simulink model "EKF_Sim_MLE"  (R2018a)
settings: Solver=ode4  StartTime=0  StopTime=time_end  FixedStep=time_step  MaxStep=0.1  RelTol=1e-15  AbsTol=1e-15
values from neighbouring files (symbols this model uses):
  mu = 398600.4418    [FFNAV_EKF_STM.m]
  N_window = 30    [FFNAV_EKF_MLE_Run.m]
  time_step = 1    [FFNAV_EKF_MLE_Run.m]
undefined symbols (not defined in the file or in its folder): a_chaser, a_target, AoP_chaser, AoP_target, e_chaser, e_target, GPS_r_STD, GPS_v_STD, i_chaser, i_target, n, Q0, R0, RAAN_chaser, RAAN_target, theta0_chaser, theta0_target
libraries: dspindex x2
settings Model: Creator=corytfraser  LastModifiedBy=Cory
settings SolverCC: AutoScaleAbsTol=off
settings DataIOCC: LimitDataPoints=on  SaveFormat=Array  SignalLoggingSaveFormat=ModelDataLogs
settings OptimizationCC: BlockReduction=off  BooleanDataType=off  ExpressionDepthLimit=2147483647  LifeSpan=inf
settings DebuggingCC: SaveWithParameterizedLinksMsg=none  UnderspecifiedInitializationDetection=Classic  MergeDetectMultiDrivingBlocksExec=none  SignalResolutionControl=TryResolveAllWithWarning  MultiTaskDSMMsg=warning  MultiTaskCondExecSysMsg=none  FcnCallInpInsideContextMsg=warning  AllowSymbolicDim=off  StateNameClashWarn=warning  SFUnexpectedBacktrackingDiag=warning  SFNoUnconditionalDefaultTransitionDiag=warning  SFExecutionAtInitializationDiag=none
settings HardwareCC: ProdBitPerPointer=32  ProdBitPerSizeT=32  ProdBitPerPtrDiffT=32  ProdLargestAtomicFloat=None  ProdIntDivRoundTo=Undefined  ProdEndianess=Unspecified  ProdWordSize=32  ProdHWDeviceType=32-bit Generic  TargetUnknown=on
settings ModelReferenceCC: PropagateSignalLabelsOutOfModel=off
settings CodeAppCC: StateflowObjectComments=on
settings GRTTargetCC: TargetLangStandard=C89/C90 (ANSI)  GeneratePreprocessorConditionals=Disable all
settings ConfigComp: CovMetricSettings=dw  CovHtmlReporting=on  CovSaveCumulativeToWorkspaceVar=on  CovSaveSingleToWorkspaceVar=on  CovExternalEMLEnable=off  CovSFcnEnable=off

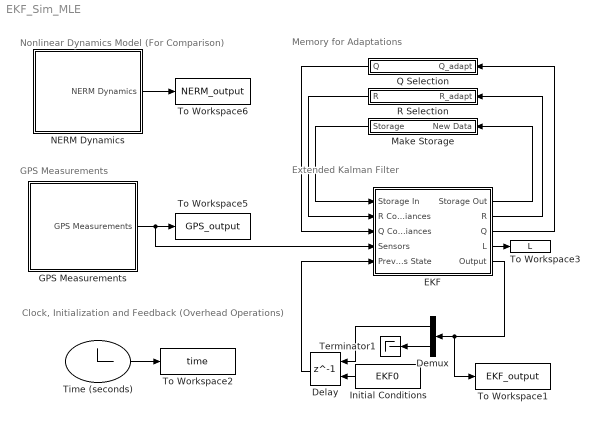
== system EKF_Sim_MLE ==
  note: Memory for Adaptations
  note: Clock, Initialization and Feedback (Overhead Operations)
  note: Extended Kalman Filter
  note: GPS Measurements
  note: Nonlinear Dynamics Model (For Comparison)
  Delay : Delay  DelayLength=1  InitialConditionSource=Input port  InitialCondition=0  SampleTime=time_step
      settings: InputPortMap=u0,p4
  Demux : Demux  Outputs=[117 -1]
  EKF : Subsystem
  "GPS Measurements " : Subsystem
      mask Display: image('C:\Users\Cory\OneDrive\FFNAV Project\MATLAB Code\NERM EKF Simulation\Masks\GPS Image.jpg');
  Initial Conditions : FromWorkspace  VariableName=EKF0  SampleTime=time_step
  Make Storage : Subsystem
  NERM Dynamics : Subsystem
      mask Display: image('C:\Users\Cory\OneDrive\FFNAV Project\MATLAB Code\NERM EKF Simulation\Masks\Proba-3.jpg');
  Q Selection : Subsystem
  R Selection : Subsystem
  Terminator1 : Terminator
  Time (seconds) : Clock
  To Workspace1 : ToWorkspace  VariableName=EKF_output  SampleTime=-1
  To Workspace2 : ToWorkspace  VariableName=time  SampleTime=-1
  To Workspace3 : ToWorkspace  VariableName=L  SampleTime=-1
  To Workspace5 : ToWorkspace  VariableName=GPS_output  SampleTime=-1
  To Workspace6 : ToWorkspace  VariableName=NERM_output  SampleTime=-1
  wires:
  Time (seconds)/1 -> To Workspace2/1
  Demux/1 -> Delay/1
  NERM Dynamics/1(NERM Dynamics) -> To Workspace6/1
  Initial Conditions/1 -> Delay/2
  Delay/1 -> EKF/5(Previous State)
  Demux/2 -> Terminator1/1
  EKF/4(L) -> To Workspace3/1
  "GPS Measurements "/1(GPS Measurements) -> EKF/4(Sensors), To Workspace5/1
  EKF/3(Q) -> Q Selection/1(Q_adapt)
  Q Selection/1(Q) -> EKF/3(Q Covariances)
  EKF/2(R) -> R Selection/1(R_adapt)
  R Selection/1(R) -> EKF/2(R Covariances)
  EKF/5(Output) -> Demux/1, To Workspace1/1
  EKF/1(Storage Out) -> Make Storage/1(New Data)
  Make Storage/1(Storage) -> EKF/1(Storage In)

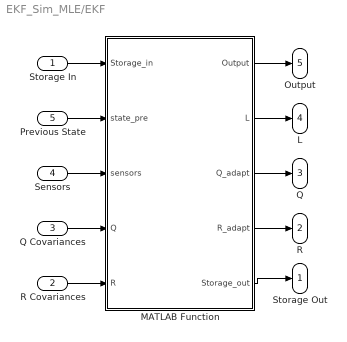
== system EKF_Sim_MLE/EKF ==
  Storage In : Inport
  R Covariances : Inport  Port=2
  Q Covariances : Inport  Port=3
  Sensors : Inport  Port=4
  Previous State : Inport  Port=5
  MATLAB Function : MATLAB Function  TreatAsAtomicUnit=on
  Storage Out : Outport
  R : Outport  Port=2
  Q : Outport  Port=3
  L : Outport  Port=4
  Output : Outport  Port=5
  wires:
  MATLAB Function/1(Output) -> Output/1
  Previous State/1 -> MATLAB Function/2(state_pre)
  Q Covariances/1 -> MATLAB Function/4(Q)
  R Covariances/1 -> MATLAB Function/5(R)
  Sensors/1 -> MATLAB Function/3(sensors)
  MATLAB Function/2(L) -> L/1
  MATLAB Function/3(Q_adapt) -> Q/1
  MATLAB Function/4(R_adapt) -> R/1
  MATLAB Function/5(Storage_out) -> Storage Out/1
  Storage In/1 -> MATLAB Function/1(Storage_in)

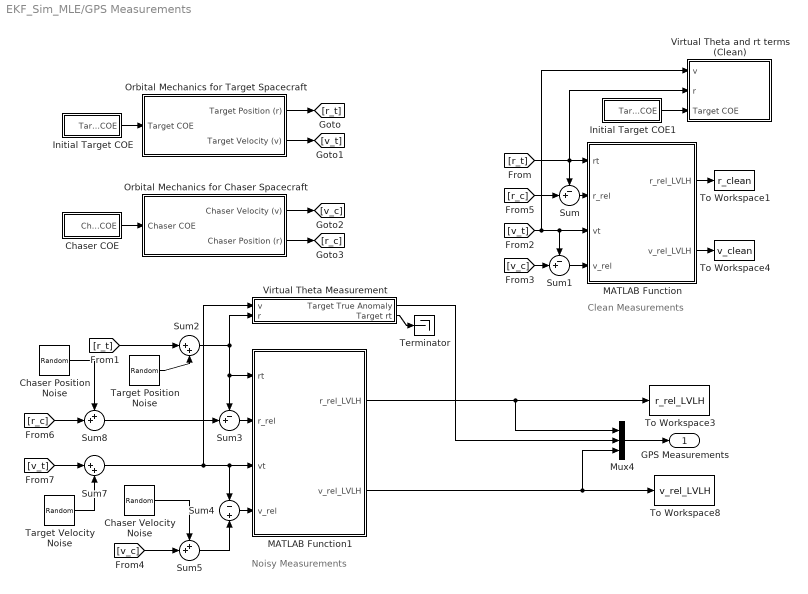
== system EKF_Sim_MLE/GPS Measurements  ==
  note: Noisy Measurements
  note: Clean Measurements
  Chaser COE : Subsystem
  Chaser Position Noise : RandomNumber  Variance=GPS_r_STD^2  Seed=1222  SampleTime=time_step
  Chaser Velocity Noise : RandomNumber  Variance=GPS_v_STD^2  Seed=99999999  SampleTime=time_step
  Initial Target COE : Subsystem
  Initial Target COE1 : Subsystem
  MATLAB Function : MATLAB Function  TreatAsAtomicUnit=on
  MATLAB Function1 : MATLAB Function  TreatAsAtomicUnit=on
  Mux4 : Mux  Inputs=3
  Orbital Mechanics for Target Spacecraft : Subsystem
  Orbital Mechanics for Chaser Spacecraft : Subsystem
  Sum : Sum  Inputs=-+|
  Sum1 : Sum  Inputs=-+|
  Sum2 : Sum  Inputs=|++
  Sum3 : Sum  Inputs=-+|
  Sum4 : Sum  Inputs=-|+
  Sum5 : Sum  Inputs=++|
  Sum7 : Sum  Inputs=|++
  Sum8 : Sum  Inputs=++|
  Target Position Noise : RandomNumber  Variance=GPS_r_STD^2  Seed=999  SampleTime=time_step
  Target Velocity Noise : RandomNumber  Variance=GPS_v_STD^2  Seed=2000  SampleTime=time_step
  Terminator : Terminator
  To Workspace1 : ToWorkspace  VariableName=r_clean  SampleTime=-1
  To Workspace3 : ToWorkspace  VariableName=r_rel_LVLH  SampleTime=-1
  To Workspace4 : ToWorkspace  VariableName=v_clean  SampleTime=-1
  To Workspace8 : ToWorkspace  VariableName=v_rel_LVLH  SampleTime=-1
  Virtual Theta Measurement : Subsystem
  Virtual Theta and rt terms (Clean) : Subsystem
  GPS Measurements : Outport
  wires:
  Orbital Mechanics for Target Spacecraft/1(Target Position (r)) -> [r_t]
  Sum/1 -> MATLAB Function/2(r_rel)
  Sum1/1 -> MATLAB Function/4(v_rel)
  MATLAB Function/2(v_rel_LVLH) -> To Workspace4/1
  MATLAB Function/1(r_rel_LVLH) -> To Workspace1/1
  Mux4/1 -> GPS Measurements/1
  Initial Target COE/1(Target COE) -> Orbital Mechanics for Target Spacecraft/1(Target COE)
  Chaser COE/1(Chaser COE) -> Orbital Mechanics for Chaser Spacecraft/1(Chaser COE)
  MATLAB Function1/2(v_rel_LVLH) -> Mux4/3, To Workspace8/1
  MATLAB Function1/1(r_rel_LVLH) -> Mux4/1, To Workspace3/1
  Sum7/1 -> Virtual Theta Measurement/1(v), MATLAB Function1/3(vt), Sum4/1
  Sum3/1 -> MATLAB Function1/2(r_rel)
  Sum4/1 -> MATLAB Function1/4(v_rel)
  Sum5/1 -> Sum4/2
  Sum8/1 -> Sum3/2
  [r_t] -> Virtual Theta and rt terms (Clean)/2(r), MATLAB Function/1(rt), Sum/1
  [v_t] -> Virtual Theta and rt terms (Clean)/1(v), Sum1/1, MATLAB Function/3(vt)
  [v_c] -> Sum1/2
  Orbital Mechanics for Chaser Spacecraft/1(Chaser Velocity (v)) -> [v_c]
  [r_c] -> Sum/2
  Orbital Mechanics for Chaser Spacecraft/2(Chaser Position (r)) -> [r_c]
  Orbital Mechanics for Target Spacecraft/2(Target Velocity (v)) -> [v_t]
  [r_t] -> Sum2/1
  [r_c] -> Sum8/2
  [v_t] -> Sum7/1
  [v_c] -> Sum5/2
  Sum2/1 -> MATLAB Function1/1(rt), Sum3/1, Virtual Theta Measurement/2(r)
  Chaser Position Noise/1 -> Sum8/1
  Target Position Noise/1 -> Sum2/2
  Target Velocity Noise/1 -> Sum7/2
  Chaser Velocity Noise/1 -> Sum5/1
  Initial Target COE1/1(Target COE) -> Virtual Theta and rt terms (Clean)/3(Target COE)
  Virtual Theta Measurement/1(Target True Anomaly) -> Mux4/2
  Virtual Theta Measurement/2(Target rt) -> Terminator/1

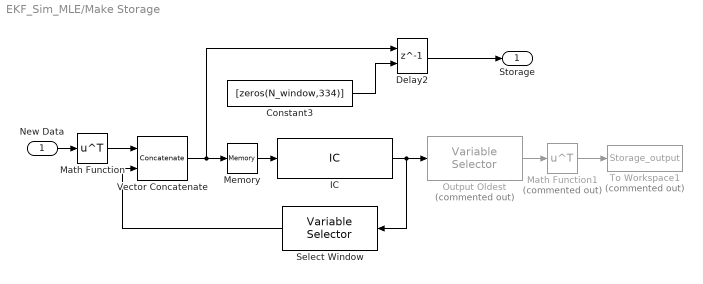
== system EKF_Sim_MLE/Make Storage ==
  New Data : Inport
  Constant3 : Constant  Value=[zeros(N_window,334)]
  Delay2 : Delay  DelayLength=1  InitialConditionSource=Input port  InitialCondition=0  SampleTime=time_step
      settings: InputPortMap=u0,p4
  IC : InitialCondition  Value=[zeros(N_window,334)]
  Math Function : Math  Operator=transpose  SaturateOnIntegerOverflow=on
  Math Function1 : Math  Commented=on  Operator=transpose  SaturateOnIntegerOverflow=on
  Memory : Memory
  Output Oldest : dspindex/Variable Selector  Commented=on  NumInputs=1  rowsOrCols=Rows  IdxMode=Fixed  Elements=N_window  ZerOneIdxMode=One-based  errmode=Clip Index  FillMode=on  FillValues=0
  Select Window : dspindex/Variable Selector  NumInputs=1  rowsOrCols=Rows  IdxMode=Fixed  Elements=1:N_window-1  ZerOneIdxMode=One-based  errmode=Clip Index  FillMode=on  FillValues=0
  To Workspace1 : ToWorkspace  Commented=on  VariableName=Storage_output  SampleTime=-1
  Vector Concatenate : Concatenate  Mode=Multidimensional array
  Storage : Outport
  wires:
  IC/1 -> Output Oldest/1, Select Window/1
  Memory/1 -> IC/1
  Select Window/1 -> Vector Concatenate/2
  New Data/1 -> Math Function/1
  Vector Concatenate/1 -> Delay2/1, Memory/1
  Math Function/1 -> Vector Concatenate/1
  Delay2/1 -> Storage/1
  Constant3/1 -> Delay2/2
  Math Function1/1 -> To Workspace1/1
  Output Oldest/1 -> Math Function1/1

== system EKF_Sim_MLE/NERM Dynamics ==
  Demux : Demux  Outputs=[10 -1]
  Demux1 : Demux  Outputs=10
  Initial Conditions : FromWorkspace  VariableName=EKF0  SampleTime=time_step
  Mux : Mux  Inputs=10
  NERM Propagation : Subsystem
  Terminator1 : Terminator
  NERM Dynamics : Outport
  wires:
  Demux1/9 -> NERM Propagation/9(theta_dot0)
  Demux1/6 -> NERM Propagation/6(x_dot0_chaser)
  Demux1/10 -> NERM Propagation/10(rt_dot0)
  Demux1/4 -> NERM Propagation/4(theta0_target)
  Demux1/3 -> NERM Propagation/3(z0_chaser)
  Initial Conditions/1 -> Demux/1
  Demux1/7 -> NERM Propagation/7(y_dot0_chaser)
  Demux1/2 -> NERM Propagation/2(y0_chaser)
  Demux1/1 -> NERM Propagation/1(x0_chaser)
  NERM Propagation/1(x) -> Mux/1
  Demux1/5 -> NERM Propagation/5(rt0)
  NERM Propagation/2(y) -> Mux/2
  NERM Propagation/3(z) -> Mux/3
  Demux/1 -> Demux1/1  "Initial  State Vector"
  NERM Propagation/7(y_dot) -> Mux/7
  NERM Propagation/4(theta_target) -> Mux/4
  NERM Propagation/9(theta_dot_target) -> Mux/9
  NERM Propagation/10(rt_dot) -> Mux/10
  NERM Propagation/6(x_dot) -> Mux/6
  NERM Propagation/8(z_dot) -> Mux/8
  NERM Propagation/5(rt) -> Mux/5
  Demux1/8 -> NERM Propagation/8(z_dot0_chaser)
  Mux/1 -> NERM Dynamics/1
  Demux/2 -> Terminator1/1

== system EKF_Sim_MLE/Q Selection ==
  Q_adapt : Inport
  Constant2 : Constant  Value=Q0
  Delay1 : Delay  DelayLength=1  InitialConditionSource=Input port  InitialCondition=0  SampleTime=time_step
      settings: InputPortMap=u0,p4
  Switch: Q Adaptation On/Off : ManualSwitch
  To Workspace4 : ToWorkspace  VariableName=Q_output  SampleTime=-1
  Q : Outport
  wires:
  Switch: Q Adaptation On/Off/1 -> Delay1/1
  Constant2/1 -> Switch: Q Adaptation On/Off/2, Delay1/2
  Q_adapt/1 -> Switch: Q Adaptation On/Off/1
  Delay1/1 -> To Workspace4/1, Q/1

== system EKF_Sim_MLE/R Selection ==
  R_adapt : Inport
  Constant3 : Constant  Value=R0
  Delay2 : Delay  DelayLength=1  InitialConditionSource=Input port  InitialCondition=0  SampleTime=time_step
      settings: InputPortMap=u0,p4
  Switch: R Adaptation On/Off : ManualSwitch
  To Workspace7 : ToWorkspace  VariableName=R_output  SampleTime=-1
  R : Outport
  wires:
  Switch: R Adaptation On/Off/1 -> Delay2/1
  Constant3/1 -> Switch: R Adaptation On/Off/2, Delay2/2
  Delay2/1 -> R/1, To Workspace7/1
  R_adapt/1 -> Switch: R Adaptation On/Off/1

== system EKF_Sim_MLE/GPS Measurements /Chaser COE ==
  Argument of Perigee (w)1 : Constant  Value=AoP_chaser
  Eccentricity (e)1 : Constant  Value=e_chaser
  Inclination (i)1 : Constant  Value=i_chaser
  Mux1 : Mux  Inputs=6
  RAAN (Omega)1 : Constant  Value=RAAN_chaser
  Semi-Major Axis (a)1 : Constant  Value=a_chaser
  True Anomaly (theta) : Constant  Value=theta0_chaser
  Chaser COE : Outport
  wires:
  Mux1/1 -> Chaser COE/1
  Argument of Perigee (w)1/1 -> Mux1/6
  True Anomaly (theta)/1 -> Mux1/1
  Semi-Major Axis (a)1/1 -> Mux1/2
  Inclination (i)1/1 -> Mux1/4
  RAAN (Omega)1/1 -> Mux1/5
  Eccentricity (e)1/1 -> Mux1/3

== system EKF_Sim_MLE/GPS Measurements /Initial Target COE ==
  Argument of Perigee (w) : Constant  Value=AoP_target
  Eccentricity (e) : Constant  Value=e_target
  Inclination (i) : Constant  Value=i_target
  Mux : Mux  Inputs=6
  RAAN (Omega) : Constant  Value=RAAN_target
  Semi-Major Axis (a) : Constant  Value=a_target
  Target True Anomaly (theta) : Constant  Value=theta0_target
  Target COE : Outport
  wires:
  Argument of Perigee (w)/1 -> Mux/6
  RAAN (Omega)/1 -> Mux/5
  Eccentricity (e)/1 -> Mux/3
  Semi-Major Axis (a)/1 -> Mux/2
  Target True Anomaly (theta)/1 -> Mux/1
  Inclination (i)/1 -> Mux/4
  Mux/1 -> Target COE/1

== system EKF_Sim_MLE/GPS Measurements /Initial Target COE1 ==
  Argument of Perigee (w) : Constant  Value=AoP_target
  Eccentricity (e) : Constant  Value=e_target
  Inclination (i) : Constant  Value=i_target
  Mux : Mux  Inputs=6
  RAAN (Omega) : Constant  Value=RAAN_target
  Semi-Major Axis (a) : Constant  Value=a_target
  Target True Anomaly (theta) : Constant  Value=theta0_target
  Target COE : Outport
  wires:
  Argument of Perigee (w)/1 -> Mux/6
  RAAN (Omega)/1 -> Mux/5
  Eccentricity (e)/1 -> Mux/3
  Semi-Major Axis (a)/1 -> Mux/2
  Target True Anomaly (theta)/1 -> Mux/1
  Inclination (i)/1 -> Mux/4
  Mux/1 -> Target COE/1

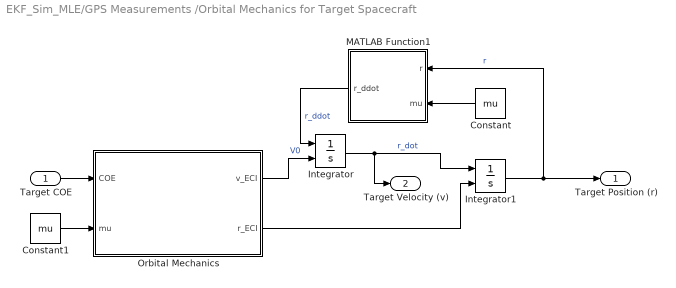
== system EKF_Sim_MLE/GPS Measurements /Orbital Mechanics for Target Spacecraft ==
  Target COE : Inport
  Constant : Constant  Value=mu
  Constant1 : Constant  Value=mu
  Integrator : Integrator  InitialConditionSource=external
  Integrator1 : Integrator  InitialConditionSource=external
  MATLAB Function1 : MATLAB Function  TreatAsAtomicUnit=on
  Orbital Mechanics : MATLAB Function  TreatAsAtomicUnit=on
  Target Position (r) : Outport
  Target Velocity (v) : Outport  Port=2
  wires:
  Integrator/1 -> Target Velocity (v)/1, Integrator1/1  "r_dot"
  MATLAB Function1/1(r_ddot) -> Integrator/1  "r_ddot"
  Integrator1/1 -> Target Position (r)/1, MATLAB Function1/1(r)  "r"
  Orbital Mechanics/2(r_ECI) -> Integrator1/2
  Orbital Mechanics/1(v_ECI) -> Integrator/2  "V0"
  Target COE/1 -> Orbital Mechanics/1(COE)
  Constant/1 -> MATLAB Function1/2(mu)
  Constant1/1 -> Orbital Mechanics/2(mu)

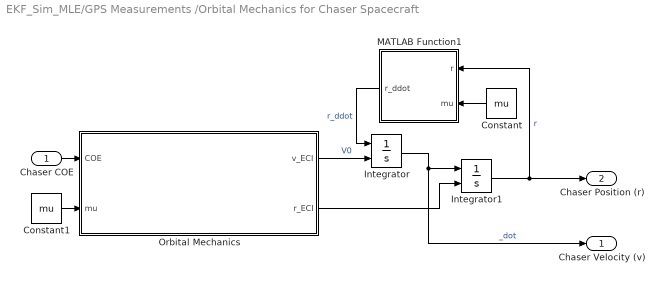
== system EKF_Sim_MLE/GPS Measurements /Orbital Mechanics for Chaser Spacecraft ==
  Chaser COE : Inport
  Constant : Constant  Value=mu
  Constant1 : Constant  Value=mu
  Integrator : Integrator  InitialConditionSource=external
  Integrator1 : Integrator  InitialConditionSource=external
  MATLAB Function1 : MATLAB Function  TreatAsAtomicUnit=on
  Orbital Mechanics : MATLAB Function  TreatAsAtomicUnit=on
  Chaser Velocity (v) : Outport
  Chaser Position (r) : Outport  Port=2
  wires:
  Integrator/1 -> Chaser Velocity (v)/1, Integrator1/1  "_dot"
  MATLAB Function1/1(r_ddot) -> Integrator/1  "r_ddot"
  Integrator1/1 -> MATLAB Function1/1(r), Chaser Position (r)/1  "r"
  Orbital Mechanics/2(r_ECI) -> Integrator1/2
  Orbital Mechanics/1(v_ECI) -> Integrator/2  "V0"
  Chaser COE/1 -> Orbital Mechanics/1(COE)
  Constant/1 -> MATLAB Function1/2(mu)
  Constant1/1 -> Orbital Mechanics/2(mu)

== system EKF_Sim_MLE/GPS Measurements /Virtual Theta Measurement ==
  v : Inport
  r : Inport  Port=2
  Constant3 : Constant  Value=theta0_target
  Integrator2 : Integrator  InitialConditionSource=external
  MATLAB Function2 : MATLAB Function  TreatAsAtomicUnit=on
  To Workspace5 : ToWorkspace  VariableName=theta_target  SampleTime=-1
  Target True Anomaly : Outport
  Target rt : Outport  Port=2
  wires:
  r/1 -> MATLAB Function2/1(r)
  Integrator2/1 -> Target True Anomaly/1, To Workspace5/1
  MATLAB Function2/1(theta_dot) -> Integrator2/1
  Constant3/1 -> Integrator2/2
  v/1 -> MATLAB Function2/2(v)
  MATLAB Function2/2(rt) -> Target rt/1

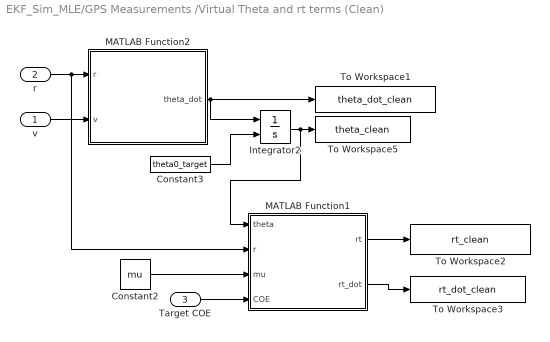
== system EKF_Sim_MLE/GPS Measurements /Virtual Theta and rt terms (Clean) ==
  v : Inport
  r : Inport  Port=2
  Target COE : Inport  Port=3
  Constant2 : Constant  Value=mu
  Constant3 : Constant  Value=theta0_target
  Integrator2 : Integrator  InitialConditionSource=external
  MATLAB Function1 : MATLAB Function  TreatAsAtomicUnit=on
  MATLAB Function2 : MATLAB Function  TreatAsAtomicUnit=on
  To Workspace1 : ToWorkspace  VariableName=theta_dot_clean  SampleTime=-1
  To Workspace2 : ToWorkspace  VariableName=rt_clean  SampleTime=-1
  To Workspace3 : ToWorkspace  VariableName=rt_dot_clean  SampleTime=-1
  To Workspace5 : ToWorkspace  VariableName=theta_clean  SampleTime=-1
  wires:
  r/1 -> MATLAB Function1/2(r), MATLAB Function2/1(r)
  Integrator2/1 -> MATLAB Function1/1(theta), To Workspace5/1
  MATLAB Function2/1(theta_dot) -> Integrator2/1, To Workspace1/1
  Constant3/1 -> Integrator2/2
  v/1 -> MATLAB Function2/2(v)
  MATLAB Function1/1(rt) -> To Workspace2/1
  MATLAB Function1/2(rt_dot) -> To Workspace3/1
  Target COE/1 -> MATLAB Function1/4(COE)
  Constant2/1 -> MATLAB Function1/3(mu)

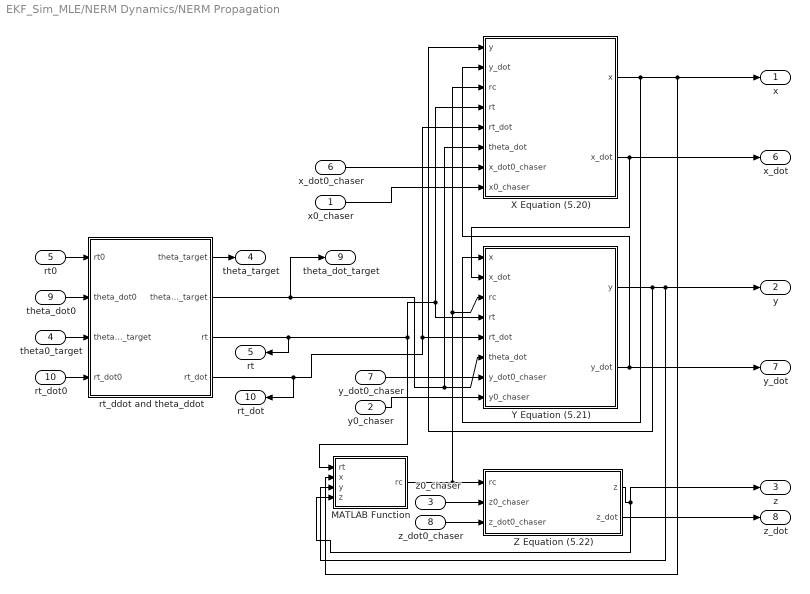
== system EKF_Sim_MLE/NERM Dynamics/NERM Propagation ==
  x0_chaser : Inport
  y0_chaser : Inport  Port=2
  z0_chaser : Inport  Port=3
  theta0_target : Inport  Port=4
  rt0 : Inport  Port=5
  x_dot0_chaser : Inport  Port=6
  y_dot0_chaser : Inport  Port=7
  z_dot0_chaser : Inport  Port=8
  theta_dot0 : Inport  Port=9
  rt_dot0 : Inport  Port=10
  MATLAB Function : MATLAB Function  TreatAsAtomicUnit=on
  X Equation (5.20) : Subsystem
  Y Equation (5.21) : Subsystem
  Z Equation (5.22) : Subsystem
  rt_ddot and theta_ddot : Subsystem
  x : Outport
  y : Outport  Port=2
  z : Outport  Port=3
  theta_target : Outport  Port=4
  rt : Outport  Port=5
  x_dot : Outport  Port=6
  y_dot : Outport  Port=7
  z_dot : Outport  Port=8
  theta_dot_target : Outport  Port=9
  rt_dot : Outport  Port=10
  wires:
  MATLAB Function/1(rc) -> X Equation (5.20)/3(rc), Y Equation (5.21)/3(rc), Z Equation (5.22)/1(rc)
  rt_ddot and theta_ddot/4(rt_dot) -> X Equation (5.20)/5(rt_dot), Y Equation (5.21)/5(rt_dot), rt_dot/1
  Y Equation (5.21)/2(y_dot) -> y_dot/1, X Equation (5.20)/2(y_dot)
  X Equation (5.20)/2(x_dot) -> x_dot/1, Y Equation (5.21)/2(x_dot)
  rt_ddot and theta_ddot/2(theta_dot_target) -> theta_dot_target/1, X Equation (5.20)/6(theta_dot), Y Equation (5.21)/6(theta_dot)
  rt_ddot and theta_ddot/3(rt) -> Y Equation (5.21)/4(rt), X Equation (5.20)/4(rt), MATLAB Function/1(rt), rt/1
  X Equation (5.20)/1(x) -> x/1, MATLAB Function/2(x), Y Equation (5.21)/1(x)
  Y Equation (5.21)/1(y) -> y/1, MATLAB Function/3(y), X Equation (5.20)/1(y)
  Z Equation (5.22)/1(z) -> MATLAB Function/4(z), z/1
  rt0/1 -> rt_ddot and theta_ddot/1(rt0)
  theta_dot0/1 -> rt_ddot and theta_ddot/2(theta_dot0)
  y_dot0_chaser/1 -> Y Equation (5.21)/7(y_dot0_chaser)
  y0_chaser/1 -> Y Equation (5.21)/8(y0_chaser)
  x0_chaser/1 -> X Equation (5.20)/8(x0_chaser)
  x_dot0_chaser/1 -> X Equation (5.20)/7(x_dot0_chaser)
  z0_chaser/1 -> Z Equation (5.22)/2(z0_chaser)
  z_dot0_chaser/1 -> Z Equation (5.22)/3(z_dot0_chaser)
  theta0_target/1 -> rt_ddot and theta_ddot/3(theta0_target)
  rt_dot0/1 -> rt_ddot and theta_ddot/4(rt_dot0)
  Z Equation (5.22)/2(z_dot) -> z_dot/1
  rt_ddot and theta_ddot/1(theta_target) -> theta_target/1

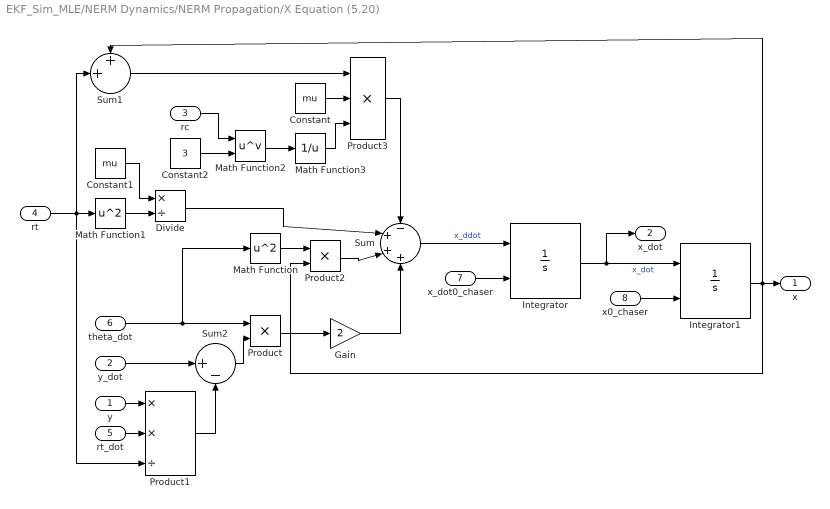
== system EKF_Sim_MLE/NERM Dynamics/NERM Propagation/X Equation (5.20) ==
  y : Inport
  y_dot : Inport  Port=2
  rc : Inport  Port=3
  rt : Inport  Port=4
  rt_dot : Inport  Port=5
  theta_dot : Inport  Port=6
  x_dot0_chaser : Inport  Port=7
  x0_chaser : Inport  Port=8
  Constant : Constant  Value=mu
  Constant1 : Constant  Value=mu
  Constant2 : Constant  Value=3
  Divide : Product  Inputs=*/
  Gain : Gain  Gain=2
  Integrator : Integrator  InitialConditionSource=external
  Integrator1 : Integrator  InitialConditionSource=external
  Math Function : Math  Operator=square  SaturateOnIntegerOverflow=on
  Math Function1 : Math  Operator=square  SaturateOnIntegerOverflow=on
  Math Function2 : Math  Operator=pow  SaturateOnIntegerOverflow=on
  Math Function3 : Math  Operator=reciprocal  SaturateOnIntegerOverflow=on
  Product : Product
  Product1 : Product  Inputs=**/
  Product2 : Product
  Product3 : Product  Inputs=3
  Sum : Sum  Inputs=-+++
  Sum1 : Sum  Inputs=++|
  Sum2 : Sum  Inputs=|+-
  x : Outport
  x_dot : Outport  Port=2
  wires:
  Sum/1 -> Integrator/1  "x_ddot"
  Integrator/1 -> Integrator1/1, x_dot/1  "x_dot"
  x_dot0_chaser/1 -> Integrator/2
  Constant/1 -> Product3/2
  Integrator1/1 -> Product2/2, Sum1/1, x/1
  rc/1 -> Math Function2/1
  x0_chaser/1 -> Integrator1/2
  rt/1 -> Sum1/2, Product1/3, Math Function1/1
  Sum1/1 -> Product3/1
  Constant1/1 -> Divide/1
  Divide/1 -> Sum/2
  Product/1 -> Gain/1
  theta_dot/1 -> Product/1, Math Function/1
  y_dot/1 -> Sum2/1
  y/1 -> Product1/1
  rt_dot/1 -> Product1/2
  Product1/1 -> Sum2/2
  Sum2/1 -> Product/2
  Math Function/1 -> Product2/1
  Product2/1 -> Sum/3
  Gain/1 -> Sum/4
  Math Function1/1 -> Divide/2
  Constant2/1 -> Math Function2/2
  Math Function2/1 -> Math Function3/1
  Math Function3/1 -> Product3/3
  Product3/1 -> Sum/1

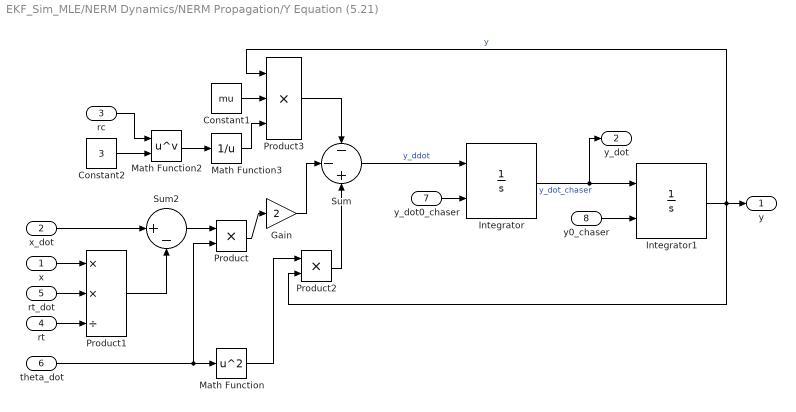
== system EKF_Sim_MLE/NERM Dynamics/NERM Propagation/Y Equation (5.21) ==
  x : Inport
  x_dot : Inport  Port=2
  rc : Inport  Port=3
  rt : Inport  Port=4
  rt_dot : Inport  Port=5
  theta_dot : Inport  Port=6
  y_dot0_chaser : Inport  Port=7
  y0_chaser : Inport  Port=8
  Constant1 : Constant  Value=mu
  Constant2 : Constant  Value=3
  Gain : Gain  Gain=2
  Integrator : Integrator  InitialConditionSource=external
  Integrator1 : Integrator  InitialConditionSource=external
  Math Function : Math  Operator=square  SaturateOnIntegerOverflow=on
  Math Function2 : Math  Operator=pow  SaturateOnIntegerOverflow=on
  Math Function3 : Math  Operator=reciprocal  SaturateOnIntegerOverflow=on
  Product : Product
  Product1 : Product  Inputs=**/
  Product2 : Product
  Product3 : Product  Inputs=3
  Sum : Sum  Inputs=--+
  Sum2 : Sum  Inputs=|+-
  y : Outport
  y_dot : Outport  Port=2
  wires:
  y_dot0_chaser/1 -> Integrator/2
  y0_chaser/1 -> Integrator1/2
  Integrator/1 -> y_dot/1, Integrator1/1  "y_dot_chaser"
  Sum/1 -> Integrator/1  "y_ddot"
  Integrator1/1 -> Product2/2, Product3/1, y/1  "y"
  Product/1 -> Gain/1
  theta_dot/1 -> Product/2, Math Function/1
  Product1/1 -> Sum2/2
  Math Function/1 -> Product2/1
  Gain/1 -> Sum/2
  Product2/1 -> Sum/3
  x_dot/1 -> Sum2/1
  x/1 -> Product1/1
  rt_dot/1 -> Product1/2
  rt/1 -> Product1/3
  Sum2/1 -> Product/1
  Constant1/1 -> Product3/2
  rc/1 -> Math Function2/1
  Constant2/1 -> Math Function2/2
  Math Function2/1 -> Math Function3/1
  Math Function3/1 -> Product3/3
  Product3/1 -> Sum/1

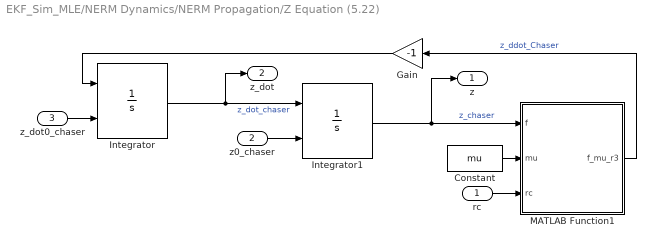
== system EKF_Sim_MLE/NERM Dynamics/NERM Propagation/Z Equation (5.22) ==
  rc : Inport
  z0_chaser : Inport  Port=2
  z_dot0_chaser : Inport  Port=3
  Constant : Constant  Value=mu
  Gain : Gain  Gain=-1
  Integrator : Integrator  InitialConditionSource=external
  Integrator1 : Integrator  InitialConditionSource=external
  MATLAB Function1 : MATLAB Function  TreatAsAtomicUnit=on
  z : Outport
  z_dot : Outport  Port=2
  wires:
  Constant/1 -> MATLAB Function1/2(mu)
  Integrator/1 -> z_dot/1, Integrator1/1  "z_dot_chaser"
  Integrator1/1 -> z/1, MATLAB Function1/1(f)  "z_chaser"
  Gain/1 -> Integrator/1
  MATLAB Function1/1(f_mu_r3) -> Gain/1  "z_ddot_Chaser"
  z_dot0_chaser/1 -> Integrator/2
  z0_chaser/1 -> Integrator1/2
  rc/1 -> MATLAB Function1/3(rc)

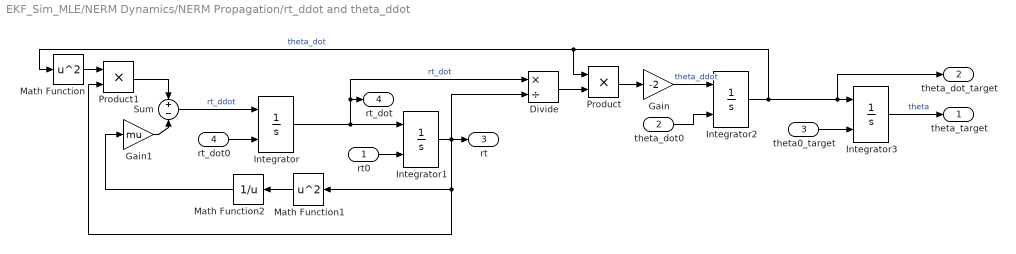
== system EKF_Sim_MLE/NERM Dynamics/NERM Propagation/rt_ddot and theta_ddot ==
  rt0 : Inport
  theta_dot0 : Inport  Port=2
  theta0_target : Inport  Port=3
  rt_dot0 : Inport  Port=4
  Divide : Product  Inputs=*/
  Gain : Gain  Gain=-2
  Gain1 : Gain  Gain=mu
  Integrator : Integrator  InitialConditionSource=external
  Integrator1 : Integrator  InitialConditionSource=external
  Integrator2 : Integrator  InitialConditionSource=external  InitialCondition=n
  Integrator3 : Integrator  InitialConditionSource=external
  Math Function : Math  Operator=square  SaturateOnIntegerOverflow=on
  Math Function1 : Math  Operator=square  SaturateOnIntegerOverflow=on
  Math Function2 : Math  Operator=reciprocal  SaturateOnIntegerOverflow=on
  Product : Product
  Product1 : Product
  Sum : Sum  Inputs=+|-
  theta_target : Outport
  theta_dot_target : Outport  Port=2
  rt : Outport  Port=3
  rt_dot : Outport  Port=4
  wires:
  Gain1/1 -> Sum/2
  Math Function2/1 -> Gain1/1
  Math Function1/1 -> Math Function2/1
  Math Function/1 -> Product1/1
  Integrator3/1 -> theta_target/1  "theta"
  Product/1 -> Gain/1
  Sum/1 -> Integrator/1  "rt_ddot"
  Integrator2/1 -> Integrator3/1, theta_dot_target/1, Math Function/1, Product/1  "theta_dot"
  Integrator1/1 -> Product1/2, Math Function1/1, Divide/2, rt/1
  Integrator/1 -> Integrator1/1, Divide/1, rt_dot/1  "rt_dot"
  Divide/1 -> Product/2
  Gain/1 -> Integrator2/1  "theta_ddot"
  theta0_target/1 -> Integrator3/2
  rt_dot0/1 -> Integrator/2
  rt0/1 -> Integrator1/2
  Product1/1 -> Sum/1
  theta_dot0/1 -> Integrator2/2

== matlab function EKF_Sim_MLE/GPS Measurements /Orbital Mechanics for Target Spacecraft/MATLAB Function1 ==
  data: r input; r_ddot output; mu input
function r_ddot = r_ddot(r, mu)
% ========================================================================
% Description: This function calculates -mu/r^3 *r to propagate the radius
% vector of the orbital motion

r_ddot = -(mu/(norm(r))^3)*r;

end
% ========================================================================

== matlab function EKF_Sim_MLE/GPS Measurements /Orbital Mechanics for Target Spacecraft/Orbital Mechanics ==
  data: v_ECI output; COE input; r_ECI output; mu input
 function [v_ECI,r_ECI] = Orb_Mech(COE, mu)
% ========================================================================
% Description: This funciton calculates the initial r and v vectors, 
% given the provided classiclal orbital elements defined in the
% initialization of the simulation.

%%========================================================================
%Extract COE values
theta       = COE(1);
a           = COE(2);
e           = COE(3);
i           = COE(4);
RAAN        = COE(5);
w           = COE(6);

%%========================================================================
r   = a*(1-e^2)/(1+e*cos(theta));                               %Defining the radius (Eq. 2.32)
p   = a*(1-e^2);                                                %Defining the semilatus rectum (Eq. 2.31)
r_P = [r*cos(theta) r*sin(theta) 0]';                           %(r in perifocal frame - Eq. 2.86) 
v_P = [-sqrt(mu/p)*sin(theta) sqrt(mu/p)*(e+cos(theta)) 0]';    %(v in perifocal frame - Eq. 2.87)

%Rotation Matrix from P to ECI Frame
C_IP = [    cos(RAAN)*cos(w)-sin(RAAN)*cos(i)*sin(w) -cos(RAAN)*sin(w)-sin(RAAN)*cos(i)*cos(w) sin(RAAN)*sin(i);
            sin(RAAN)*cos(w)+cos(RAAN)*cos(i)*sin(w) -sin(RAAN)*sin(w)+cos(RAAN)*cos(i)*cos(w) -cos(RAAN)*sin(i);
                        sin(i)*sin(w)                            sin(i)*cos(w)                       cos(i)  ];

%Definition of ECI Frame
x_ECI   = [1 0 0];
y_ECI   = [0 1 0];
z_ECI   = [0 0 1];
F_ECI   = [x_ECI; y_ECI; z_ECI]; %Reference Frame ECI

%r and v vectors in ECI Frame
r_ECI   = F_ECI*C_IP*r_P;
v_ECI   = F_ECI*C_IP*v_P;

%z_vec_ECI  = cross(r_ECI, v_ECI)/norm(cross(r_ECI, v_ECI));    %Check orientation of z vector
%X_ECI      = [r_ECI v_ECI]';                                   %State Vector in ECI components (Eq. 2.82)

r_mag = norm(r_ECI);
r_hat = r_ECI/r_mag;

end
% ========================================================================

== matlab function EKF_Sim_MLE/GPS Measurements /Orbital Mechanics for Chaser Spacecraft/MATLAB Function1 ==
  data: r input; r_ddot output; mu input
function r_ddot = r_ddot(r, mu)
% ========================================================================
% Description: This function calculates -mu/r^3 *r to propagate the radius
% vector of the orbital motion

r_ddot = -(mu/(norm(r))^3)*r;

end
% ========================================================================

== matlab function EKF_Sim_MLE/GPS Measurements /Orbital Mechanics for Chaser Spacecraft/Orbital Mechanics ==
  data: v_ECI output; COE input; r_ECI output; mu input
function [v_ECI,r_ECI] = Orb_Mech(COE, mu)
% ========================================================================
% Description: This funciton calculates the initial r and v vectors, 
% given the provided classiclal orbital elements defined in the
% initialization of the simulation.

%%========================================================================
%Extract COE values
theta       = COE(1);
a           = COE(2);
e           = COE(3);
i           = COE(4);
RAAN        = COE(5);
w           = COE(6);

%%========================================================================
r   = a*(1-e^2)/(1+e*cos(theta));                               %Defining the radius (Eq. 2.32)
p   = a*(1-e^2);                                                %Defining the semilatus rectum (Eq. 31)
r_P = [r*cos(theta) r*sin(theta) 0]';                           %(r in perifocal frame - Eq. 2.86) 
v_P = [-sqrt(mu/p)*sin(theta) sqrt(mu/p)*(e+cos(theta)) 0]';    %(v in perifocal frame - Eq. 2.87)

%Rotation Matrix from P to ECI Frame
C_IP = [    cos(RAAN)*cos(w)-sin(RAAN)*cos(i)*sin(w) -cos(RAAN)*sin(w)-sin(RAAN)*cos(i)*cos(w) sin(RAAN)*sin(i);
            sin(RAAN)*cos(w)+cos(RAAN)*cos(i)*sin(w) -sin(RAAN)*sin(w)+cos(RAAN)*cos(i)*cos(w) -cos(RAAN)*sin(i);
                        sin(i)*sin(w)                            sin(i)*cos(w)                       cos(i)  ];

%Definition of ECI Frame
x_ECI   = [1 0 0];
y_ECI   = [0 1 0];
z_ECI   = [0 0 1];
F_ECI   = [x_ECI; y_ECI; z_ECI]; %Reference Frame ECI

%r and v vectors in ECI Frame
r_ECI   = F_ECI*C_IP*r_P;
v_ECI   = F_ECI*C_IP*v_P;

%z_vec_ECI  = cross(r_ECI, v_ECI)/norm(cross(r_ECI, v_ECI));    %Check orientation of z vector
%X_ECI      = [r_ECI v_ECI]';                                   %State Vector in ECI components (Eq. 2.82)

r_mag = norm(r_ECI);
r_hat = r_ECI/r_mag;

end
% ========================================================================

== matlab function EKF_Sim_MLE/GPS Measurements /MATLAB Function ==
  data: rt input; r_rel input; vt input; r_rel_LVLH output; v_rel input; v_rel_LVLH output
 function [r_rel_LVLH, v_rel_LVLH] = To_LVLH(rt, r_rel, vt, v_rel)
% =========================================================================
% Description: This function converts the relative r and v from ECI Frame
% to LVLH Frame by applying the appropriate rotation matrices.
% =========================================================================
%Determine unit vectors for LVLH Frame
Lx      = rt/norm(rt);
Lz      = cross(rt, vt)/norm(cross(rt, vt));
Ly      = cross(Lz, Lx);

%Align unit vectors into rows
Lx      = Lx';
Ly      = Ly';
Lz      = Lz';

%Arranging vectrix for LVLH Frame
F_LVLH  = [ Lx      
            Ly
            Lz ];

%ECI Frame is defined as such
F_ECI   = [ 1 0 0 
            0 1 0
            0 0 1 ];
     
%Compute roration matrix - ECI to LVLH
C_LI    = F_LVLH*F_ECI';

%Computing relative velocity in LVLH frame, accounting for rotation 
omega =  cross(rt,vt)/norm(rt)^2;
v_rel = v_rel - cross(omega,r_rel);

%Apply rotation to obtain relative LVLH parameters
r_rel_LVLH = C_LI*r_rel; 
v_rel_LVLH = C_LI*v_rel;

end
% =========================================================================

== matlab function EKF_Sim_MLE/NERM Dynamics/NERM Propagation/MATLAB Function ==
  data: rt input; x input; y input; z input; rc output
function rc = calc_rc(rt, x, y, z)
% ========================================================================
% Description: This function calculates the radius of the chaser given the
% x, y z and rt components

%Inputs:
%    rt = Target Radius
%    x = Chaser relative x position
%    y = Chaser relative y position
%    z = Chaser relative z position
%Outputs:
%    rc = Chaser Radius

rc = sqrt((rt+x)^2+y^2+z^2);
end
% ========================================================================

== matlab function EKF_Sim_MLE/NERM Dynamics/NERM Propagation/Z Equation (5.22)/MATLAB Function1 ==
  data: f input; f_mu_r3 output; mu input; rc input
function f_mu_r3 = mu_rc3(f, mu, rc)
% ========================================================================
% Description: This function calculates mu/rc^3 and multiplies it with the
% incoming signal for the z equation of motion.

f_mu_r3 = (mu/rc^3)*f;
end
% ========================================================================

== matlab function EKF_Sim_MLE/GPS Measurements /Virtual Theta Measurement/MATLAB Function2 ==
  data: r input; v input; theta_dot output; rt output
function [theta_dot, rt] = theta_dot(r, v)
% ========================================================================
% Description: This function calculates h/r^2 to propagate the true 
% anomaly of the target spacecraft
rt = norm(r);
h = norm(cross(r,v));
theta_dot = h/rt^2;

end
% ========================================================================

== matlab function EKF_Sim_MLE/GPS Measurements /MATLAB Function1 ==
  data: rt input; r_rel input; vt input; r_rel_LVLH output; v_rel input; v_rel_LVLH output
 function [r_rel_LVLH, v_rel_LVLH] = To_LVLH(rt, r_rel, vt, v_rel)
% =========================================================================
% Description: This function converts the relative r and v from ECI Frame
% to LVLH Frame by applying the appropriate rotation matrices.
% =========================================================================
%Determine unit vectors for LVLH Frame
Lx      = rt/norm(rt);
Lz      = cross(rt, vt)/norm(cross(rt, vt));
Ly      = cross(Lz, Lx);

%Align unit vectors into rows
Lx      = Lx';
Ly      = Ly';
Lz      = Lz';

%Arranging vectrix for LVLH Frame
F_LVLH  = [ Lx
            Ly
            Lz ];

%ECI Frame is defined as such
F_ECI   = [ 1 0 0 
            0 1 0
            0 0 1 ];
     
%Compute roration matrix - ECI to LVLH
C_LI    = F_LVLH*F_ECI';

%Computing relative velocity in LVLH frame, accounting for rotation 
omega =  cross(rt,vt)/norm(rt)^2;
v_rel = v_rel - cross(omega,r_rel);

%Apply rotation to obtain relative LVLH parameters
r_rel_LVLH = C_LI*r_rel; 
v_rel_LVLH = C_LI*v_rel;

end
% =========================================================================

== matlab function EKF_Sim_MLE/GPS Measurements /Virtual Theta and rt terms (Clean)/MATLAB Function2 ==
  data: r input; v input; theta_dot output
function theta_dot  = theta_dot(r, v)
% ========================================================================
% Description: This function calculates h/r^2 to propagate the true 
% anomaly of the target spacecraft
rt = norm(r);
h = norm(cross(r,v));
theta_dot = h/rt^2;

end
% ========================================================================

== matlab function EKF_Sim_MLE/EKF/MATLAB Function ==
  data: Storage_in input; state_pre input; sensors input; Output output; Q input; R input; L output; Q_adapt output; R_adapt output; Storage_out output; time_step parameter; mu parameter
 function [Output, L, Q_adapt, R_adapt, Storage_out] = USE_EKF_MLE(Storage_in,state_pre, sensors, Q, R, time_step, mu)
%% USE_EKF ===============================================================
% ========================================================================
% Description: This function calls the FFNAV_EKF Function, which completes 
% the covariance propagation and correction phases of the EKF algorithm. 
% The output is then passed back to the simulink model.

Output = zeros(243,1);
Storage_out = zeros(334,1);
Q_adapt = zeros(10,10);
R_adapt = zeros(7,7);
[Output, Storage_out, L, Q_adapt, R_adapt] = FFNAV_EKF_MLE(Storage_in,time_step, mu, state_pre, sensors, Q, R);
end
% ========================================================================

== matlab function EKF_Sim_MLE/GPS Measurements /Virtual Theta and rt terms (Clean)/MATLAB Function1 ==
  data: theta input; r input; rt output; rt_dot output; mu input; COE input
function [rt, rt_dot]  = rt_rtdot(theta, r, mu, COE)
% ========================================================================
% Description: This function calculates h/r^2 to propagate the true 
% anomaly of the target spacecraft

theta0       = COE(1);
a           = COE(2);
e           = COE(3);
i           = COE(4);
RAAN        = COE(5);
w           = COE(6);

rt      = norm(r);
p       = a*(1-e^2);
rt_dot  = sqrt(mu/p)*e*sin(theta);

end
% ========================================================================
